simulink model "CDMA_test"  (Simulink 7.7)
settings: Solver=FixedStepDiscrete  StartTime=0.0  StopTime=50  RelTol=1e-3
values from neighbouring files (symbols this model uses):
  D = [  1 -1  1 -1  1  1 -1 -1 ... (first row only)    [cdma.m]    (also in compressed_sampling.m = idct(eye(5000,5000)))
libraries: commrandsrc2 x6, commfilt2 x2
settings Model: Creator=ArunKB  LastModifiedBy=ArunKB

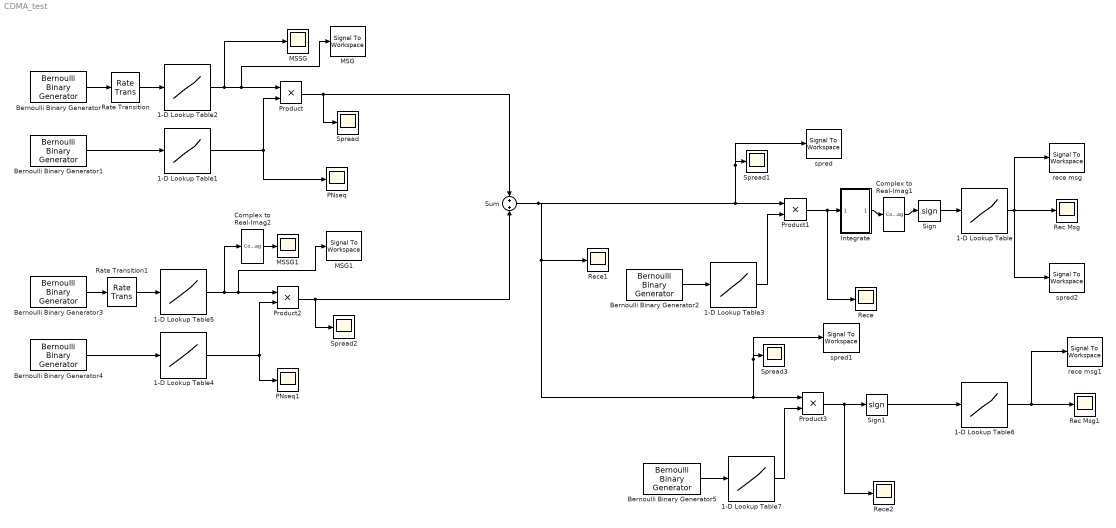
== system CDMA_test ==
  1-D Lookup Table : Lookup_n-D  NumberOfTableDimensions=1  BreakpointsForDimension1=[-1,0,1]  Table=[-1,-1,1]  RndMeth=Simplest  InputSameDT=on
  1-D Lookup Table{1..5,7} (6 alike) : Lookup_n-D  NumberOfTableDimensions=1  BreakpointsForDimension1=[0 1]  Table=[-1 1]  RndMeth=Simplest  InputSameDT=on
  1-D Lookup Table6 : Lookup_n-D  NumberOfTableDimensions=1  BreakpointsForDimension1=[-1,0,1]  Table=[-1,-1,1]  RndMeth=Simplest  InputSameDT=on
  Bernoulli Binary Generator : commrandsrc2/Bernoulli Binary Generator  SystemSampleTime=-1  P=0.5  seed=randseed  Ts=1  frameBased=off  sampPerFrame=1  orient=off  outDataType=double
  Bernoulli Binary Generator1 : commrandsrc2/Bernoulli Binary Generator  SystemSampleTime=-1  P=0.5  seed=88  Ts=.01  frameBased=off  sampPerFrame=1  orient=off  outDataType=double
  Bernoulli Binary Generator2 : commrandsrc2/Bernoulli Binary Generator  SystemSampleTime=-1  P=0.5  seed=45  Ts=.01  frameBased=off  sampPerFrame=1  orient=off  outDataType=double
  Bernoulli Binary Generator3 : commrandsrc2/Bernoulli Binary Generator  SystemSampleTime=-1  P=0.5  seed=randseed  Ts=1  frameBased=off  sampPerFrame=1  orient=off  outDataType=double
  Bernoulli Binary Generator4 : commrandsrc2/Bernoulli Binary Generator  SystemSampleTime=-1  P=0.5  seed=45  Ts=.01  frameBased=off  sampPerFrame=1  orient=off  outDataType=double
  Bernoulli Binary Generator5 : commrandsrc2/Bernoulli Binary Generator  SystemSampleTime=-1  P=0.5  seed=88  Ts=.01  frameBased=off  sampPerFrame=1  orient=off  outDataType=double
  Complex to Real-Imag1 : ComplexToRealImag  Output=Real
  Complex to Real-Imag2 : ComplexToRealImag  Output=Real
  Integrate : Subsystem
  MSG : SignalToWorkspace  VariableName=msg  SaveFormat=Array  Save2DMode=2-D array (concatenate along first dimension)
      settings: CopyFcn=dspblkcopystw(gcbh);
  MSG1 : SignalToWorkspace  VariableName=msg1  SaveFormat=Array  Save2DMode=2-D array (concatenate along first dimension)
      settings: CopyFcn=dspblkcopystw(gcbh);
  MSSG : Scope
  MSSG1 : Scope
      settings: SaveName=ScopeData6
  PNseq : Scope
      settings: SaveName=ScopeData2
  PNseq1 : Scope
      settings: SaveName=ScopeData7
  Product{,1..3} (4 alike) : Product  RndMeth=Zero
  Rate Transition : RateTransition
  Rate Transition1 : RateTransition
  Rec Msg : Scope
      settings: SaveName=ScopeData4
  Rec Msg1 : Scope
      settings: SaveName=ScopeData10
  Rece : Scope
      settings: SaveName=ScopeData3
  Rece1 : Scope
      settings: SaveName=ScopeData9
  Rece2 : Scope
      settings: SaveName=ScopeData11
  Sign : Signum
  Sign1 : Signum
  Spread{,1..3} (4 alike) : Scope
      Spread1 settings: SaveName=ScopeData5
      Spread2 settings: SaveName=ScopeData8
      Spread3 settings: SaveName=ScopeData12
  Sum : Sum  Inputs=+|+
  rece msg : SignalToWorkspace  VariableName=rece  SaveFormat=Array  Save2DMode=2-D array (concatenate along first dimension)
      settings: CopyFcn=dspblkcopystw(gcbh);
  rece msg1 : SignalToWorkspace  VariableName=rece1  SaveFormat=Array  Save2DMode=2-D array (concatenate along first dimension)
      settings: CopyFcn=dspblkcopystw(gcbh);
  spred : SignalToWorkspace  VariableName=spread  SaveFormat=Array  Save2DMode=2-D array (concatenate along first dimension)
      settings: CopyFcn=dspblkcopystw(gcbh);
  spred1 : SignalToWorkspace  VariableName=spread1  SaveFormat=Array  Save2DMode=2-D array (concatenate along first dimension)
      settings: CopyFcn=dspblkcopystw(gcbh);
  spred2 : SignalToWorkspace  VariableName=spread2  SaveFormat=Array  Save2DMode=2-D array (concatenate along first dimension)
      settings: CopyFcn=dspblkcopystw(gcbh);
  wires:
  1-D Lookup Table2/1 -> Product/1, MSG/1, MSSG/1
  Rate Transition/1 -> 1-D Lookup Table2/1
  1-D Lookup Table1/1 -> Product/2, PNseq/1
  Bernoulli Binary Generator/1 -> Rate Transition/1
  1-D Lookup Table3/1 -> Product1/2
  Product1/1 -> Rece/1, Integrate/1(In1)
  1-D Lookup Table/1 -> spred2/1, rece msg/1, Rec Msg/1
  Sign/1 -> 1-D Lookup Table/1
  1-D Lookup Table5/1 -> Product2/1, MSG1/1, Complex to Real-Imag2/1
  1-D Lookup Table4/1 -> PNseq1/1, Product2/2
  Bernoulli Binary Generator3/1 -> Rate Transition1/1
  Sum/1 -> Product1/1, Spread1/1, spred/1, Rece1/1, spred1/1, Spread3/1, Product3/1
  Bernoulli Binary Generator1/1 -> 1-D Lookup Table1/1
  Product/1 -> Sum/1, Spread/1
  Product2/1 -> Sum/2, Spread2/1
  1-D Lookup Table7/1 -> Product3/2
  Product3/1 -> Sign1/1, Rece2/1
  1-D Lookup Table6/1 -> Rec Msg1/1, rece msg1/1
  Sign1/1 -> 1-D Lookup Table6/1
  Bernoulli Binary Generator5/1 -> 1-D Lookup Table7/1
  Complex to Real-Imag1/1 -> Sign/1
  Integrate/1(Out1) -> Complex to Real-Imag1/1
  Complex to Real-Imag2/1 -> MSSG1/1
  Bernoulli Binary Generator2/1 -> 1-D Lookup Table3/1
  Bernoulli Binary Generator4/1 -> 1-D Lookup Table4/1
  Rate Transition1/1 -> 1-D Lookup Table5/1

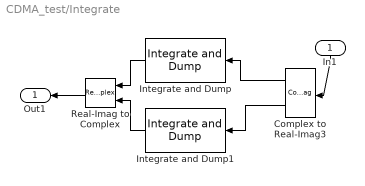
== system CDMA_test/Integrate ==
  In1 : Inport
  Complex to Real-Imag3 : ComplexToRealImag
  Integrate and Dump : commfilt2/Integrate and Dump  obssamples=20  offsetsamples=0  nodump=off  roundingMode=Floor  overflowMode=off
  Integrate and Dump1 : commfilt2/Integrate and Dump  obssamples=20  offsetsamples=0  nodump=off  roundingMode=Floor  overflowMode=off
  Real-Imag to Complex : RealImagToComplex
  Out1 : Outport
  wires:
  Complex to Real-Imag3/1 -> Integrate and Dump/1
  Complex to Real-Imag3/2 -> Integrate and Dump1/1
  Integrate and Dump/1 -> Real-Imag to Complex/1
  Integrate and Dump1/1 -> Real-Imag to Complex/2
  In1/1 -> Complex to Real-Imag3/1
  Real-Imag to Complex/1 -> Out1/1
